simulink model "arduinouno_drive_closedloop"  (R2017a)
settings: Solver=ode3  StartTime=0.0  StopTime=inf  RelTol=1e-3  EnableMultiTasking=on
PreLoadFcn:
  | k_synchronize=2;
InitFcn:
  | k_synchronize=2;
  | lego_drive_closedloop_InitData.mdl = get_param(bdroot,'Name');
  | lego_drive_closedloop_InitData.cs = getActiveConfigSet(lego_drive_closedloop_InitData.mdl);
undefined symbols (not defined in the file): serial
libraries: arduinolib x10, simulink x2, instrumentlib x2, realtime_examples_misc x1
PreSaveFcn:
  | set_param(gcs, 'Location',[35 56 895 605])
CloseFcn:
  | clear k_synchronize lego_drive_closedloop_InitData
settings Model: ExtModeTrigDuration=2  Creator=The MathWorks Inc.  LastModifiedBy=hemma
settings DataIOCC: LimitDataPoints=on  SaveFormat=Array  SignalLoggingSaveFormat=ModelDataLogs
settings OptimizationCC: PassReuseOutputArgsAs=Individual arguments  ExpressionDepthLimit=2147483647  MaxStackSize=64
settings DebuggingCC: UnderspecifiedInitializationDetection=Classic  MergeDetectMultiDrivingBlocksExec=none  InheritedTsInSrcMsg=none  ParameterPrecisionLossMsg=none  ParameterTunabilityLossMsg=error  FcnCallInpInsideContextMsg=warning  StateNameClashWarn=warning  SFUnexpectedBacktrackingDiag=warning  SFNoUnconditionalDefaultTransitionDiag=warning  SFExecutionAtInitializationDiag=none
settings HardwareCC: ProdBitPerInt=16  ProdBitPerPointer=16  ProdBitPerSizeT=16  ProdBitPerPtrDiffT=16  ProdLargestAtomicFloat=None  ProdWordSize=8  ProdHWDeviceType=Atmel->AVR
settings ModelReferenceCC: PropagateSignalLabelsOutOfModel=off
settings SFSimCC: MATLABDynamicMemAlloc=off
settings RTWCC: SystemTargetFile=ert.tlc  HardwareBoard=Arduino Uno  TLCOptions=-aInlineSetEventsForThisBaseRateFcn=TLC_FALSE -aSuppressMultiTaskScheduler=TLC_FALSE -aRateBasedStepFcn=1  TemplateMakefile=ert_default_tmf  Description=Embedded Coder  GenerateReport=on  RTWVerbose=off  Toolchain=Arduino AVR  BuildConfiguration=Faster Runs  IncludeHyperlinkInReport=on  LaunchReport=on  GenerateTraceInfo=on  GenerateTraceReport=on  GenerateTraceReportSl=on  GenerateTraceReportSf=on  GenerateTraceReportEml=on
settings CodeAppCC: ForceParamTrailComments=on  IgnoreCustomStorageClasses=off  OperatorAnnotations=on  SimulinkDataObjDesc=on  SFDataObjDesc=on  MATLABFcnDesc=on  CustomSymbolStrType=$N$R$M  InsertBlockDesc=on  MATLABSourceComments=on  InternalIdentifier=Classic
settings ERTTargetCC: SupportContinuousTime=on  SupportVariableSizeSignals=on
settings ConfigComp: CovMetricSettings=dw  CovHtmlReporting=on  CovSaveCumulativeToWorkspaceVar=on  CovSaveSingleToWorkspaceVar=on  CovExternalEMLEnable=off  CovSFcnEnable=off

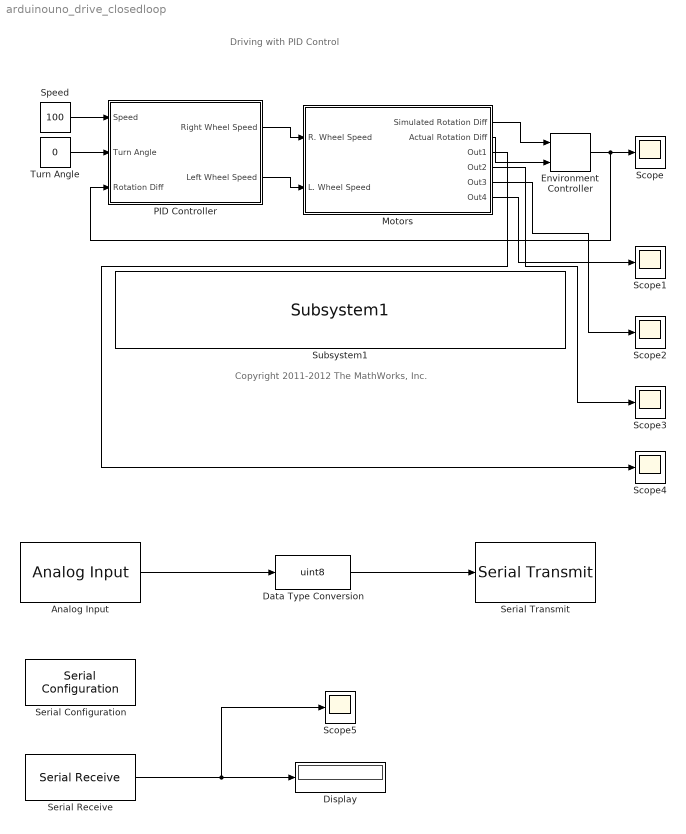
== system arduinouno_drive_closedloop ==
  note: Copyright 2011-2012 The MathWorks, Inc.
  note: Driving with PID Control
  Analog Input : arduinolib/Analog Input  pinNumber=2  sampleTime=0.1  blockPlatform=arduino
  Data Type Conversion : DataTypeConversion  OutDataTypeStr=uint8
  Display : Display
  Environment Controller : simulink/Signal Routing/Environment Controller
      settings: SourceProductName=Simulink  SourceProductBaseCode=SL
  Motors : Subsystem  VariantControl=DoSim
      settings: MinAlgLoopOccurrences=on
  PID Controller : Subsystem
  Scope{,1..5} (6 alike) : Scope
  Serial Configuration : instrumentlib/Serial Configuration  Priority=-200000  ComPortMenu=<Please select a port...>  ComPort=COM11  ObjConstructor=serial('COM11');  BaudRate=9600  DataBits=8  Parity=none  StopBits=1  FlowControl=none  Timeout=10  ByteOrder=LittleEndian
  Serial Receive : instrumentlib/Serial Receive  ComPortMenu=<Please select a port...>  ComPort=COM11  ObjConstructor=serial('COM11');  Terminator=<none>  DataSize=[1 1]  DataType=uint8  EnableBlockingMode=on  ActionDataUnavailable=Output last received value  CustomValue=0  SampleTime=0.01
  Serial Transmit : arduinolib/Serial Transmit  portNumber=0  sendmode=write  sendformat=Decimal  floatprecision=2  blockPlatform=arduino
      settings: SourceProductName=Simulink Support Package for Arduino Hardware
  Speed : Constant  Value=100  OutMin=0  OutMax=100  OutDataTypeStr=single  SampleTime=0.001
  Subsystem1 : realtime_examples_misc/Subsystem1  SystemSampleTime=-1
  Turn Angle : Constant  Value=0  OutMin=-20  OutMax=20  OutDataTypeStr=single  SampleTime=0.001
  wires:
  Speed/1 -> PID Controller/1(Speed)
  Turn Angle/1 -> PID Controller/2(Turn Angle)
  Environment Controller/1 -> Scope/1, PID Controller/3(Rotation Diff)
  PID Controller/1(Right Wheel Speed) -> Motors/1(R. Wheel Speed)
  PID Controller/2(Left Wheel Speed) -> Motors/2(L. Wheel Speed)
  Motors/1(Simulated Rotation Diff) -> Environment Controller/1
  Motors/2(Actual Rotation Diff) -> Environment Controller/2
  Motors/6(Out4) -> Scope1/1
  Motors/5(Out3) -> Scope2/1
  Motors/4(Out2) -> Scope3/1
  Motors/3(Out1) -> Scope4/1
  Analog Input/1 -> Data Type Conversion/1
  Data Type Conversion/1 -> Serial Transmit/1
  Serial Receive/1 -> Scope5/1, Display/1

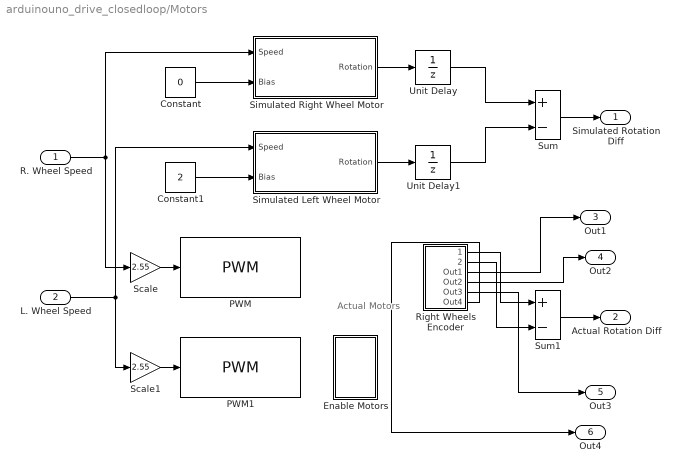
== system arduinouno_drive_closedloop/Motors ==
  note: Actual
      | Motors
  R. Wheel Speed : Inport
  L. Wheel Speed : Inport  Port=2
  Constant : Constant  Value=0  OutDataTypeStr=single
  Constant1 : Constant  Value=2  OutDataTypeStr=single
  Enable Motors : Subsystem
  PWM : arduinolib/PWM  pinNumber=10  blockPlatform=arduino
  PWM1 : arduinolib/PWM  pinNumber=11  blockPlatform=arduino
  Right Wheels Encoder : Subsystem
  Scale : Gain  Gain=2.55
  Scale1 : Gain  Gain=2.55
  Simulated Left Wheel Motor : Subsystem
  Simulated Right Wheel Motor : Subsystem
  Sum : Sum  Inputs=+-  OutDataTypeStr=Inherit: Same as first input
  Sum1 : Sum  Inputs=+-  OutDataTypeStr=Inherit: Same as first input
  Unit Delay : UnitDelay  SampleTime=-1
  Unit Delay1 : UnitDelay  SampleTime=-1
  Simulated Rotation Diff : Outport
  Actual Rotation Diff : Outport  Port=2
  Out1 : Outport  Port=3
  Out2 : Outport  Port=4
  Out3 : Outport  Port=5
  Out4 : Outport  Port=6
  wires:
  Simulated Right Wheel Motor/1(Rotation) -> Unit Delay/1
  L. Wheel Speed/1 -> Simulated Left Wheel Motor/1(Speed), Scale1/1
  Simulated Left Wheel Motor/1(Rotation) -> Unit Delay1/1
  Constant/1 -> Simulated Right Wheel Motor/2(Bias)
  Constant1/1 -> Simulated Left Wheel Motor/2(Bias)
  R. Wheel Speed/1 -> Simulated Right Wheel Motor/1(Speed), Scale/1
  Unit Delay/1 -> Sum/1
  Unit Delay1/1 -> Sum/2
  Sum/1 -> Simulated Rotation Diff/1
  Right Wheels Encoder/1(Encoder) -> Sum1/1
  Sum1/1 -> Actual Rotation Diff/1
  Scale/1 -> PWM/1
  Scale1/1 -> PWM1/1
  Right Wheels Encoder/2(Encoder1) -> Sum1/2
  Right Wheels Encoder/3(Out1) -> Out1/1
  Right Wheels Encoder/4(Out2) -> Out2/1
  Right Wheels Encoder/5(Out3) -> Out3/1
  Right Wheels Encoder/6(Out4) -> Out4/1

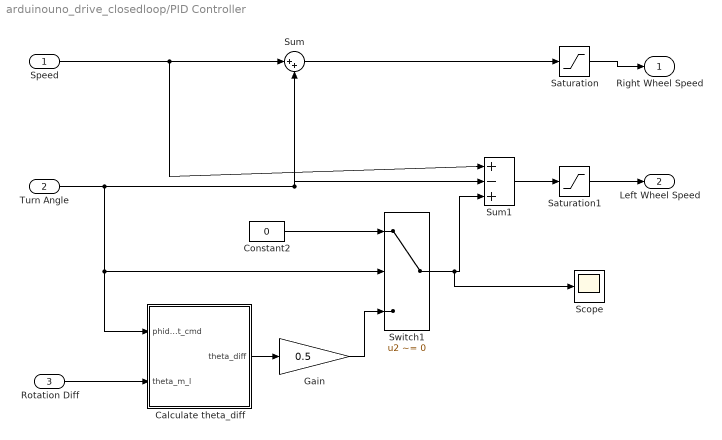
== system arduinouno_drive_closedloop/PID Controller ==
  Speed : Inport
  Turn Angle : Inport  Port=2
  Rotation Diff : Inport  Port=3
  Calculate theta_diff : Subsystem
  Constant2 : Constant  Value=0  OutDataTypeStr=single
  Gain : Gain  Gain=0.5
  Saturation : Saturate  UpperLimit=100  LowerLimit=0
      settings: AttributesFormatString=max = %<UpperLimit>\nmin = %<LowerLimit>
  Saturation1 : Saturate  UpperLimit=100  LowerLimit=0
      settings: AttributesFormatString=max = %<UpperLimit>\nmin = %<LowerLimit>
  Scope : Scope
  Sum : Sum  Inputs=|++  OutDataTypeStr=Inherit: Same as first input
  Sum1 : Sum  Inputs=|+-+  OutDataTypeStr=Inherit: Same as first input
  Switch1 : Switch  Criteria=u2 ~= 0
  Right Wheel Speed : Outport
  Left Wheel Speed : Outport  Port=2
  wires:
  Constant2/1 -> Switch1/1
  Gain/1 -> Switch1/3
  Switch1/1 -> Sum1/3, Scope/1
  Sum1/1 -> Saturation1/1
  Sum/1 -> Saturation/1
  Speed/1 -> Sum/1, Sum1/1
  Saturation/1 -> Right Wheel Speed/1
  Saturation1/1 -> Left Wheel Speed/1
  Turn Angle/1 -> Sum/2, Sum1/2, Switch1/2, Calculate theta_diff/1(phidot_cmd)
  Rotation Diff/1 -> Calculate theta_diff/2(theta_m_l)
  Calculate theta_diff/1(theta_diff) -> Gain/1

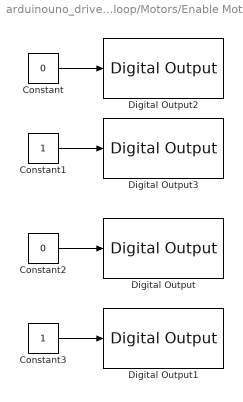
== system arduinouno_drive_closedloop/Motors/Enable Motors ==
  Constant : Constant  Value=0  OutDataTypeStr=boolean
  Constant1 : Constant  OutDataTypeStr=boolean
  Constant2 : Constant  Value=0  OutDataTypeStr=boolean
  Constant3 : Constant  OutDataTypeStr=boolean
  Digital Output : arduinolib/Digital Output  pinNumber=2  blockPlatform=arduino
  Digital Output1 : arduinolib/Digital Output  pinNumber=3  blockPlatform=arduino
  Digital Output2 : arduinolib/Digital Output  pinNumber=4  blockPlatform=arduino
  Digital Output3 : arduinolib/Digital Output  pinNumber=5  blockPlatform=arduino
  wires:
  Constant3/1 -> Digital Output1/1
  Constant2/1 -> Digital Output/1
  Constant/1 -> Digital Output2/1
  Constant1/1 -> Digital Output3/1

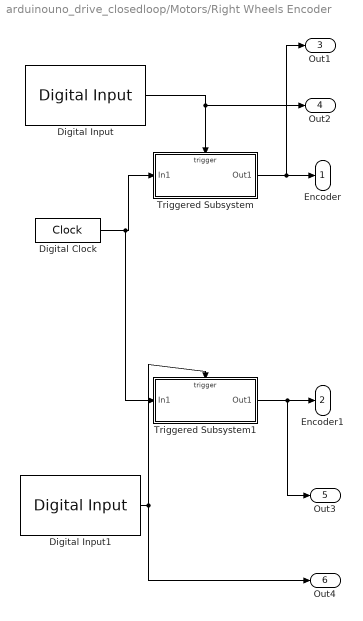
== system arduinouno_drive_closedloop/Motors/Right Wheels Encoder ==
  Digital Clock : DigitalClock  SampleTime=-1
  Digital Input : arduinolib/Digital Input  pinNumber=8  sampleTime=0.001  blockPlatform=arduino
      settings: SourceProductName=Simulink Support Package for Arduino Hardware
  Digital Input1 : arduinolib/Digital Input  pinNumber=9  sampleTime=0.001  blockPlatform=arduino
      settings: SourceProductName=Simulink Support Package for Arduino Hardware
  Triggered Subsystem : Subsystem  TreatAsAtomicUnit=on
  Triggered Subsystem1 : Subsystem  TreatAsAtomicUnit=on
  Encoder : Outport
  Encoder1 : Outport  Port=2
  Out1 : Outport  Port=3
  Out2 : Outport  Port=4
  Out3 : Outport  Port=5
  Out4 : Outport  Port=6
  wires:
  Digital Input/1 -> Triggered Subsystem/Trigger, Out2/1
  Triggered Subsystem/1(Out1) -> Out1/1, Encoder/1
  Triggered Subsystem1/1(Out1) -> Out3/1, Encoder1/1
  Digital Input1/1 -> Triggered Subsystem1/Trigger, Out4/1
  Digital Clock/1 -> Triggered Subsystem1/1(In1), Triggered Subsystem/1(In1)

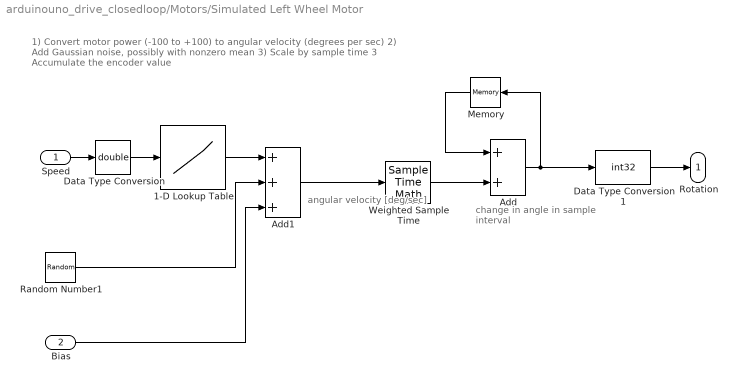
== system arduinouno_drive_closedloop/Motors/Simulated Left Wheel Motor ==
  note: 1) Convert motor power (-100 to +100) to angular velocity (degrees per sec)
      | 2) Add Gaussian noise, possibly with nonzero mean
      | 3) Scale by sample time
      | 3 Accumulate the encoder value
  note: change in angle
      | in sample interval
  note: angular velocity
      | [deg/sec]
  Speed : Inport
  Bias : Inport  Port=2
  1-D Lookup Table : Lookup_n-D  NumberOfTableDimensions=1  BreakpointsForDimension1=[-100 0 100]  Table=[-360 0 360]  ExtrapMethod=Clip  UseLastTableValue=on  RndMeth=Simplest  InputSameDT=on
  Add : Sum  AccumDataTypeStr=single  OutDataTypeStr=single
  Add1 : Sum  Inputs=+++  OutDataTypeStr=single
  Data Type Conversion : DataTypeConversion  OutDataTypeStr=double  RndMeth=Round
  Data Type Conversion1 : DataTypeConversion  OutDataTypeStr=int32
  Memory : Memory  InheritSampleTime=on  LinearizeAsDelay=on
  Random Number1 : RandomNumber  Variance=5  Seed=randi(1000)
  Weighted Sample Time : SampleTimeMath  TsampMathOp=*
  Rotation : Outport
  wires:
  1-D Lookup Table/1 -> Add1/1
  Random Number1/1 -> Add1/2
  Speed/1 -> Data Type Conversion/1
  Memory/1 -> Add/1
  Add/1 -> Memory/1, Data Type Conversion1/1
  Weighted Sample Time/1 -> Add/2
  Bias/1 -> Add1/3
  Add1/1 -> Weighted Sample Time/1
  Data Type Conversion/1 -> 1-D Lookup Table/1
  Data Type Conversion1/1 -> Rotation/1

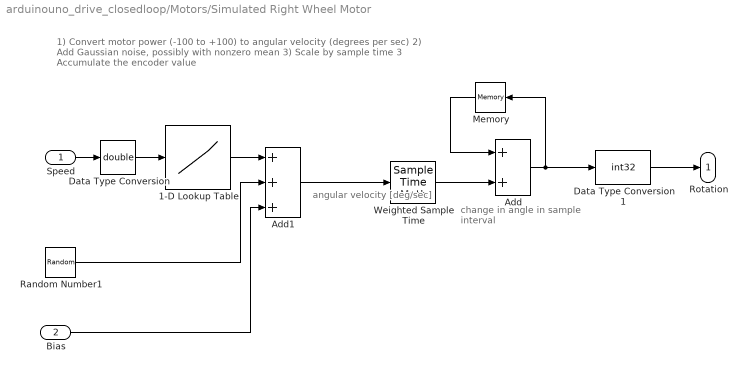
== system arduinouno_drive_closedloop/Motors/Simulated Right Wheel Motor ==
  note: change in angle
      | in sample interval
  note: angular velocity
      | [deg/sec]
  note: 1) Convert motor power (-100 to +100) to angular velocity (degrees per sec)
      | 2) Add Gaussian noise, possibly with nonzero mean
      | 3) Scale by sample time
      | 3 Accumulate the encoder value
  Speed : Inport
  Bias : Inport  Port=2
  1-D Lookup Table : Lookup_n-D  NumberOfTableDimensions=1  BreakpointsForDimension1=[-100 0 100]  Table=[-360 0 360]  ExtrapMethod=Clip  UseLastTableValue=on  RndMeth=Simplest  InputSameDT=on
  Add : Sum  OutDataTypeStr=single
  Add1 : Sum  Inputs=+++  OutDataTypeStr=single
  Data Type Conversion : DataTypeConversion  OutDataTypeStr=double  RndMeth=Round
  Data Type Conversion1 : DataTypeConversion  OutDataTypeStr=int32
  Memory : Memory  InheritSampleTime=on  LinearizeAsDelay=on
  Random Number1 : RandomNumber  Variance=5  Seed=randi(1000)
  Weighted Sample Time : SampleTimeMath  TsampMathOp=*
  Rotation : Outport
  wires:
  Data Type Conversion/1 -> 1-D Lookup Table/1
  Add1/1 -> Weighted Sample Time/1
  Bias/1 -> Add1/3
  Weighted Sample Time/1 -> Add/2
  Add/1 -> Memory/1, Data Type Conversion1/1
  Memory/1 -> Add/1
  Speed/1 -> Data Type Conversion/1
  Random Number1/1 -> Add1/2
  1-D Lookup Table/1 -> Add1/1
  Data Type Conversion1/1 -> Rotation/1

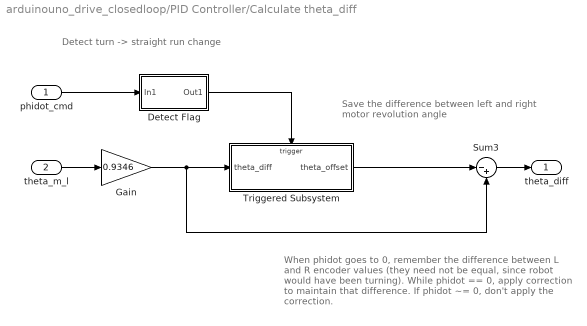
== system arduinouno_drive_closedloop/PID Controller/Calculate theta_diff ==
  note: Detect turn -> straight run change
  note: Save the difference between
      | left and right motor revolution angle
  note: When phidot goes to 0, remember the difference
      | between L and R encoder values (they need not be equal,
      | since robot would have been turning). While phidot == 0,
      | apply correction to maintain that difference.
      | If phidot ~= 0, don't apply the correction.
  phidot_cmd : Inport
  theta_m_l : Inport  Port=2
  Detect Flag : Subsystem
  Gain : Gain  Gain=0.9346  ParamDataTypeStr=single
  Sum3 : Sum  Inputs=|-+  OutDataTypeStr=Inherit: Same as first input
  Triggered Subsystem : Subsystem  TreatAsAtomicUnit=on
  theta_diff : Outport
  wires:
  phidot_cmd/1 -> Detect Flag/1(In1)
  theta_m_l/1 -> Gain/1
  Triggered Subsystem/1(theta_offset) -> Sum3/1
  Sum3/1 -> theta_diff/1
  Detect Flag/1(Out1) -> Triggered Subsystem/Trigger
  Gain/1 -> Triggered Subsystem/1(theta_diff), Sum3/2

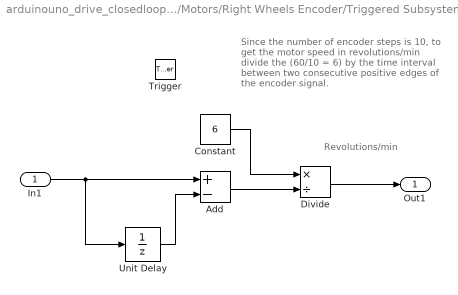
== system arduinouno_drive_closedloop/Motors/Right Wheels Encoder/Triggered Subsystem ==
  note: Revolutions/min
  note: Since the number of encoder steps is 10,
      | to get the motor speed in revolutions/min
      | divide the (60/10 = 6) by the time interval
      | between two consecutive positive edges
      | of the encoder signal.
  In1 : Inport
  Trigger : TriggerPort  VariantControl=Variant
  Add : Sum  Inputs=+-
  Constant : Constant  Value=6
  Divide : Product  Inputs=*/  OutDataTypeStr=int32
  Unit Delay : UnitDelay  SampleTime=-1
  Out1 : Outport
  wires:
  Constant/1 -> Divide/1
  Divide/1 -> Out1/1
  Add/1 -> Divide/2
  Unit Delay/1 -> Add/2
  In1/1 -> Unit Delay/1, Add/1

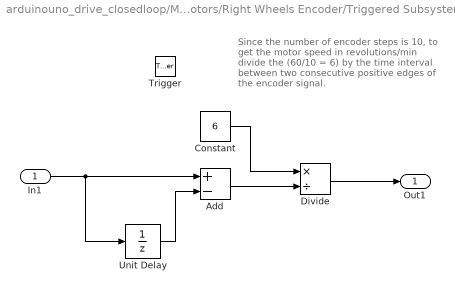
== system arduinouno_drive_closedloop/Motors/Right Wheels Encoder/Triggered Subsystem1 ==
  note: Since the number of encoder steps is 10,
      | to get the motor speed in revolutions/min
      | divide the (60/10 = 6) by the time interval
      | between two consecutive positive edges
      | of the encoder signal.
  In1 : Inport
  Trigger : TriggerPort  VariantControl=Variant
  Add : Sum  Inputs=+-
  Constant : Constant  Value=6
  Divide : Product  Inputs=*/  OutDataTypeStr=int32
  Unit Delay : UnitDelay  SampleTime=-1
  Out1 : Outport
  wires:
  In1/1 -> Add/1, Unit Delay/1
  Unit Delay/1 -> Add/2
  Add/1 -> Divide/2
  Divide/1 -> Out1/1
  Constant/1 -> Divide/1

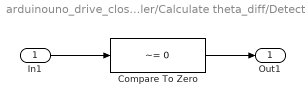
== system arduinouno_drive_closedloop/PID Controller/Calculate theta_diff/Detect Flag ==
  In1 : Inport
  Compare To Zero : simulink/Logic and Bit Operations/Compare To Zero  relop=~=  OutDataTypeStr=boolean
  Out1 : Outport
  wires:
  In1/1 -> Compare To Zero/1
  Compare To Zero/1 -> Out1/1

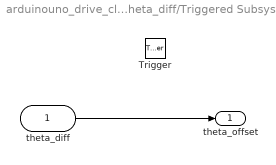
== system arduinouno_drive_closedloop/PID Controller/Calculate theta_diff/Triggered Subsystem ==
  theta_diff : Inport  LatchByDelayingOutsideSignal=on
  Trigger : TriggerPort  TriggerType=falling  VariantControl=Variant
  theta_offset : Outport
  wires:
  theta_diff/1 -> theta_offset/1
